simulink model "AB_Final_of_MPC_Bandwidth_Result_UnbalancedNew"  (R2022b)
settings: Solver=FixedStepDiscrete  StartTime=0.0  StopTime=Inf  FixedStep=100e-6  RelTol=1e-3  EnableMultiTasking=on
undefined symbols (not defined in the file): C28x, CPU1, CPU2, CurrentBypassValue, DiscIntNeverNeededParam, Down, GPTRIP1SEL, TZ1, Up
libraries: c2802xlib x20, simulink x17, dspstat3 x13, eeGeneralControl x10, c2837xDlib x5, c280xlib x5, PID_Lib x4, c2000lib x1, spsAlphaBetaZerotoabcLib x1
(part 1 of 10)
settings Model: ExtModeTrigDuration=8  Creator=user  LastModifiedBy=user
settings SolverCC: AutoInsertRateTranBlk=on
settings OptimizationCC: DefaultParameterBehavior=Inlined  DefaultUnderspecifiedDataType=single  EnhancedBackFolding=on  PassReuseOutputArgsAs=Individual arguments  MaxStackSize=1024  OptimizeBlockOrder=speed  DifferentSizesBufferReuse=on  OptimizationCustomize=off  DenormalBehavior=FlushToZero  EfficientTunableParamExpr=on
settings DebuggingCC: ParameterTunabilityLossMsg=error
settings HardwareCC: ProdBitPerChar=16  ProdBitPerInt=16  ProdBitPerPointer=32  ProdBitPerSizeT=32  ProdBitPerPtrDiffT=32  ProdLargestAtomicInteger=Integer  ProdLargestAtomicFloat=None  ProdWordSize=16  ProdLongLongMode=on  ProdHWDeviceType=Texas Instruments->C2000
settings ModelReferenceCC: ModelReferenceNumInstancesAllowed=Single
settings SFSimCC: MATLABDynamicMemAlloc=off
settings RTWCC: Description=Embedded Coder  SystemTargetFile=ert.tlc  HardwareBoard=TI Delfino F28379D LaunchPad  TLCOptions=-aInlineSetEventsForThisBaseRateFcn=TLC_FALSE -aSuppressMultiTaskScheduler=TLC_FALSE -aRateBasedStepFcn=1  TemplateMakefile=ert_default_tmf  GenerateReport=on  Toolchain=Texas Instruments Code Composer Studio (C2000)  LaunchReport=on
settings CodeAppCC: ForceParamTrailComments=on  IgnoreCustomStorageClasses=off  OperatorAnnotations=on  SimulinkDataObjDesc=on  SFDataObjDesc=on  InsertBlockDesc=on
settings ERTTargetCC: CodeReplacementLibrary=TI C28x  ExtModeTransport=4  ExtModeStaticAlloc=on  ExtModeStaticAllocSize=10000  ExtModeMexFile=ext_xcp  ExtModeIntrfLevel=Level2 - Open  InlinedParameterPlacement=NonHierarchical

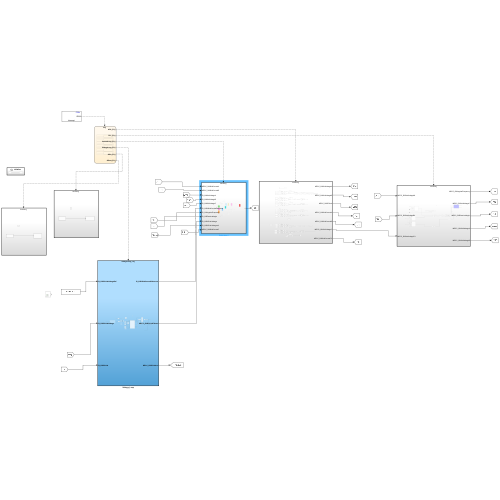
[thumbnail: Simulink's stored preview of the top-level diagram]
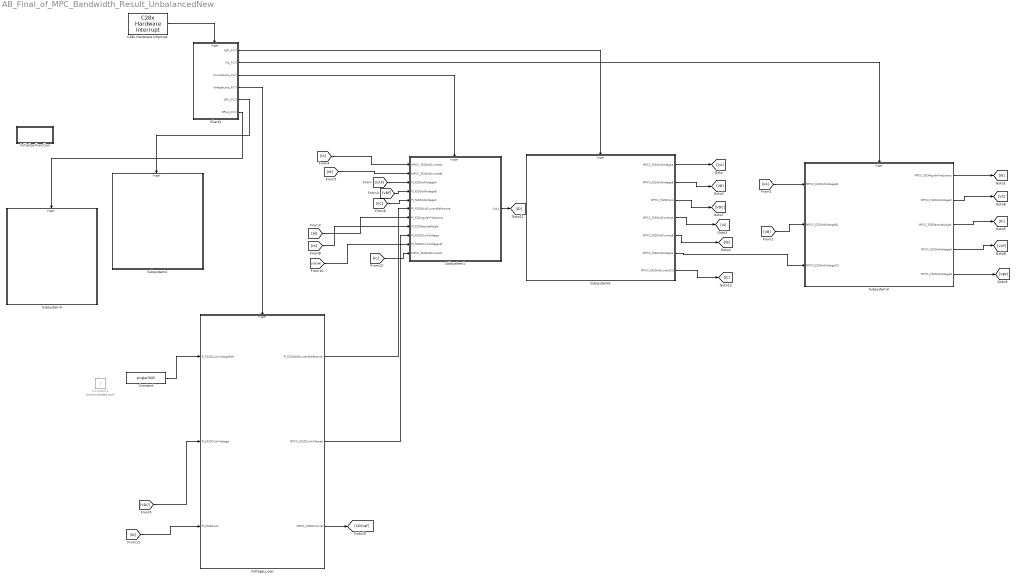
== system AB_Final_of_MPC_Bandwidth_Result_UnbalancedNew ==
  C28x Hardware Interrupt : c2000lib/Scheduling/C28x Hardware Interrupt  irqnumbers=[1]  pienumbers=[1]  irqpriorities=[1]  irqpreempts=[1]  showinput=off  dspchiptype=C280X
  Chart1 : Stateflow chart  TreatAsAtomicUnit=on
  Constant : Constant  Value=single(300)
  Constant1 : Constant  Commented=on
  Initialize Function : Subsystem  TreatAsAtomicUnit=on
  Subsystem1 : Subsystem
  Subsystem2 : Subsystem
  Subsystem3 : Subsystem
  Subsystem4 : Subsystem
  Subsystem6 : Subsystem
  Voltage_Loop : Subsystem
  wires:
  Chart1/5(GPin_FC()) -> Subsystem2/Trigger
  Chart1/3(CurrentLoop_FC()) -> Subsystem1/Trigger
  Chart1/4(VoltageLoop_FC()) -> Voltage_Loop/Trigger
  C28x Hardware Interrupt/1 -> Chart1/Trigger
  Chart1/6(GPout_FC()) -> Subsystem4/Trigger
  Chart1/2(PLL_FC()) -> Subsystem3/Trigger
  Chart1/1(ADC_FC()) -> Subsystem6/Trigger
  Subsystem3/1(MPCC_f32AngularFrequency) -> [W]
  [IA] -> Subsystem1/1(MPCC_f32GridCurrentA)
  [IB] -> Subsystem1/2(MPCC_f32GridCurrentB)
  Subsystem3/2(MPCC_f32GridVoltageC) -> [VC]
  [W] -> Subsystem1/7(PI_f32AngularFrequency)
  [th] -> Subsystem1/8(PI_f32ElectricalAngle)
  Voltage_Loop/2(MPCC_f32DCLinkFiltered) -> Subsystem1/9(PI_f32DCLinkVoltage)
  Subsystem3/3(MPCC_f32ElectricalAngle) -> [th]
  Voltage_Loop/1(PI_f32DGridCurrentReference) -> Subsystem1/6(PI_f32DGridCurrentReference)
  [VA] -> Subsystem3/1(MPCC_f32GridVoltageA2)
  [VAF] -> Subsystem1/3(PI_f32GridVoltageA)
  [VC] -> Subsystem1/5(PI_f32GridVoltageC)
  [VBF] -> Subsystem1/4(PI_f32GridVoltageB)
  Subsystem3/4(MPCC_f32GridVoltageA) -> [VAF]
  Subsystem3/5(MPCC_f32GridVoltageB) -> [VBF]
  Voltage_Loop/3(MPCC_f32DCLinkref) -> [VDCref]
  [VDCref] -> Subsystem1/10(PI_f32DCLinkVoltageref)
  [VDC] -> Voltage_Loop/2(PI_f32DCLinkVoltage)
  Constant/1 -> Voltage_Loop/1(PI_f32DCLinkVoltageRef)
  [VB] -> Subsystem3/2(MPCC_f32GridVoltageB1)
  Subsystem1/1(Out1) -> [ID]
  [ID] -> Voltage_Loop/3(PI_f32DCLink)
  Subsystem6/6(MPCC_f32GridVoltageC) -> Subsystem3/3(MPCC_f32GridVoltageC3)
  Subsystem6/7(MPCC_f32GridCurrentC3) -> [IC]
  [IC] -> Subsystem1/11(MPCC_f32GridCurrentC)
  Subsystem6/1(MPCC_f32GridVoltageA) -> [VA]
  Subsystem6/2(MPCC_f32GridVoltageB) -> [VB]
  Subsystem6/3(MPCC_f32DCLink) -> [VDC]
  Subsystem6/4(MPCC_f32GridCurrentA) -> [IA]
  Subsystem6/5(MPCC_f32GridCurrentB) -> [IB]

== system AB_Final_of_MPC_Bandwidth_Result_UnbalancedNew/Initialize Function ==
  Constant : Constant  Value=boolean(0)
  Digital Output : c2837xDlib/Digital Output  GPIO_Number=GPIO8~GPIO15  GPIO_Bit0=off  GPIO_BIT0_Toggle=off  GPIO_Bit1=off  GPIO_BIT1_Toggle=off  GPIO_Bit2=off  GPIO_BIT2_Toggle=off  GPIO_Bit3=on  GPIO_BIT3_Toggle=off  GPIO_Bit4=off  GPIO_BIT4_Toggle=off  GPIO_Bit5=off  GPIO_BIT5_Toggle=off  GPIO_Bit6=off  GPIO_BIT6_Toggle=off  GPIO_Bit7=off  GPIO_BIT7_Toggle=off
  Event Listener : EventListener  DisableCoverage=on  EventName=reset
  wires:
  Constant/1 -> Digital Output/1
